simulink model "punto2asig"  (R2021a)
settings: Solver=VariableStepAuto  StartTime=0.0  StopTime=40  RelTol=1e-3
settings Model: Creator=Daniel Rojas  LastModifiedBy=retou

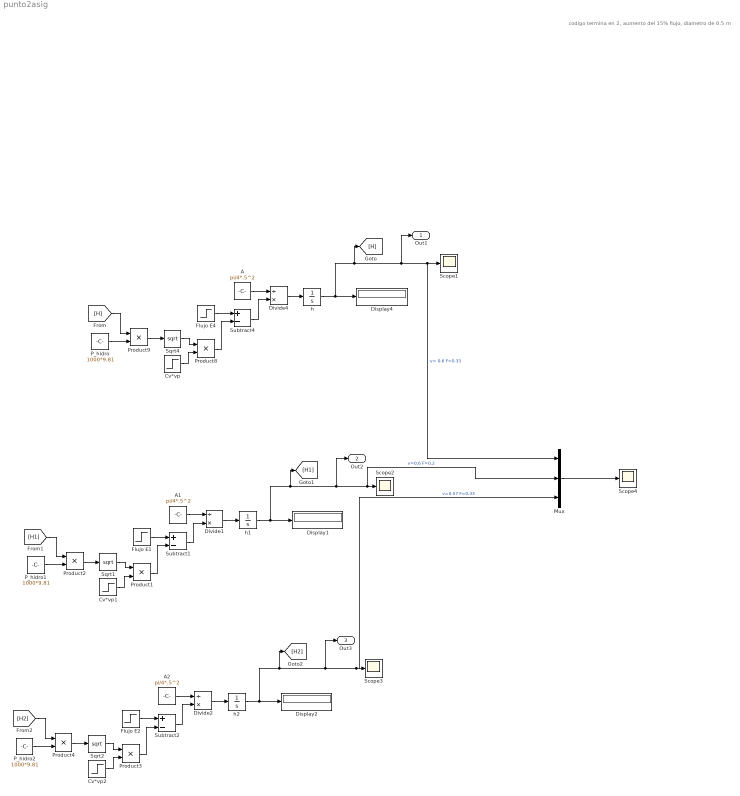
== system punto2asig ==
  note: codigo termina en 2, aumento del 15% flujo, diametro de 0.5 m
  A : Constant  Value=pi/4*.5^2
  A1 : Constant  Value=pi/4*.5^2
  A2 : Constant  Value=pi/4*.5^2
  Cv*vp : Step  Time=15  Before=0.0041*0.6  After=0.0041*0.691  SampleTime=0
  Cv*vp1 : Step  Time=15  Before=0.0041*0.6  After=0.0041*0.691  SampleTime=0
  Cv*vp2 : Step  Time=15  Before=0.0041*0.6  After=0.0041*0.57  SampleTime=0
  Display1 : Display
  Display2 : Display
  Display4 : Display
  Divide1 : Product  Inputs=/*
  Divide2 : Product  Inputs=/*
  Divide4 : Product  Inputs=/*
  Flujo E1 : Step  Time=10  Before=0.2  After=0.2*1.15  SampleTime=0
  Flujo E2 : Step  Time=10  Before=0.33  After=0.33*1.15  SampleTime=0
  Flujo E4 : Step  Time=10  Before=0.33  After=0.33*1.15  SampleTime=0
  Mux : Mux  Inputs=3
  P_hidro : Constant  Value=1000*9.81
  P_hidro1 : Constant  Value=1000*9.81
  P_hidro2 : Constant  Value=1000*9.81
  Product{1..4,8..9} (6 alike) : Product
  Scope{1..4} (4 alike) : Scope
  Sqrt1 : Sqrt  SaturateOnIntegerOverflow=on
  Sqrt2 : Sqrt  SaturateOnIntegerOverflow=on
  Sqrt4 : Sqrt  SaturateOnIntegerOverflow=on
  Subtract1 : Sum  Inputs=+-
  Subtract2 : Sum  Inputs=+-
  Subtract4 : Sum  Inputs=+-
  h : Integrator  InitialCondition=1.83  LimitOutput=on  UpperSaturationLimit=2.2  LowerSaturationLimit=0
  h1 : Integrator  InitialCondition=1.83  LimitOutput=on  UpperSaturationLimit=2.2  LowerSaturationLimit=0
  h2 : Integrator  InitialCondition=1.83  LimitOutput=on  UpperSaturationLimit=2.2  LowerSaturationLimit=0
  Out1 : Outport
  Out2 : Outport  Port=2
  Out3 : Outport  Port=3
  wires:
  Flujo E4/1 -> Subtract4/1
  P_hidro/1 -> Product9/2
  Divide4/1 -> h/1
  Product9/1 -> Sqrt4/1
  Sqrt4/1 -> Product8/1
  Cv*vp/1 -> Product8/2
  h/1 -> [H], Out1/1, Mux/1, Scope1/1, Display4/1  "v= 0.6 F=0.33"
  Subtract4/1 -> Divide4/2
  A/1 -> Divide4/1
  Product8/1 -> Subtract4/2
  [H] -> Product9/1
  [H1] -> Product2/1
  Product1/1 -> Subtract1/2
  A1/1 -> Divide1/1
  Product2/1 -> Sqrt1/1
  h1/1 -> [H1], Out2/1, Mux/2, Scope2/1, Display1/1  "v=0.6 F=0.2"
  Subtract1/1 -> Divide1/2
  Sqrt1/1 -> Product1/1
  Divide1/1 -> h1/1
  Cv*vp1/1 -> Product1/2
  P_hidro1/1 -> Product2/2
  Flujo E1/1 -> Subtract1/1
  [H2] -> Product4/1
  Product3/1 -> Subtract2/2
  A2/1 -> Divide2/1
  Product4/1 -> Sqrt2/1
  h2/1 -> [H2], Out3/1, Mux/3, Scope3/1, Display2/1  "v=0.57 F=0.33"
  Subtract2/1 -> Divide2/2
  Sqrt2/1 -> Product3/1
  Divide2/1 -> h2/1
  Cv*vp2/1 -> Product3/2
  P_hidro2/1 -> Product4/2
  Flujo E2/1 -> Subtract2/1
  Mux/1 -> Scope4/1
